simulink model "MATLAB02"  (R2023a)
settings: Solver=VariableStepAuto  StartTime=0.0  StopTime=0.1  RelTol=1e-3
libraries: spsCurrentMeasurementLib x3, spsControlledCurrentSourceLib x2, spsSeriesRLCBranchLib x2, spsDCVoltageSourceLib x1, sps_lib x1
settings Model: Creator=吉禹畅  LastModifiedBy=吉禹畅

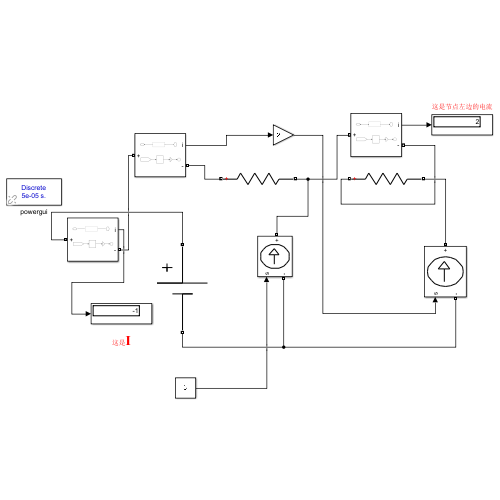
[thumbnail: Simulink's stored preview of the top-level diagram]
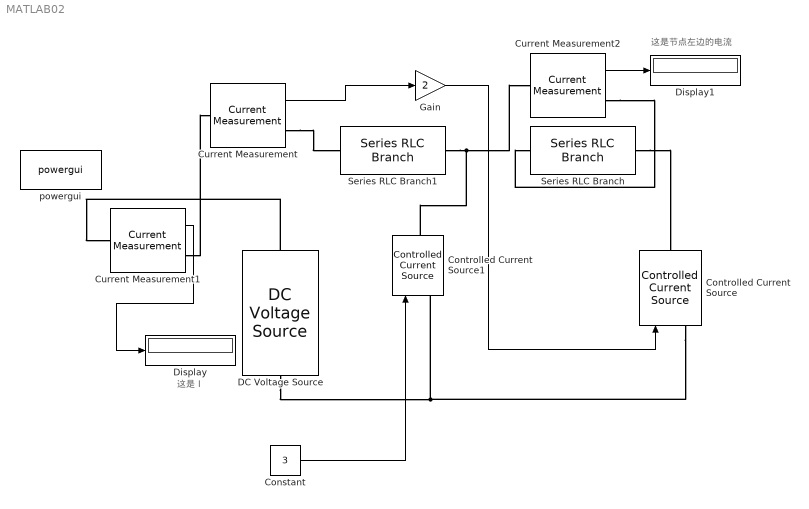
== system MATLAB02 ==
  note: 这是节点左边的电流
  note: 这是 I
  Constant : Constant  Value=3
  Controlled Current Source : spsControlledCurrentSourceLib/Controlled Current Source  Initialize=on  Source_Type=DC  Amplitude=0  Phase=0  Frequency=0  Measurements=None
  Controlled Current Source1 : spsControlledCurrentSourceLib/Controlled Current Source  Initialize=on  Source_Type=DC  Amplitude=3  Phase=0  Frequency=0  Measurements=None
  Current Measurement : spsCurrentMeasurementLib/Current Measurement  PhasorSimulation=off  OutputType=Complex  PSBequivalent=0
  Current Measurement1 : spsCurrentMeasurementLib/Current Measurement  PhasorSimulation=off  OutputType=Complex  PSBequivalent=0
  Current Measurement2 : spsCurrentMeasurementLib/Current Measurement  PhasorSimulation=off  OutputType=Complex  PSBequivalent=0
  DC Voltage Source : spsDCVoltageSourceLib/DC Voltage Source  Amplitude=10  Measurements=None
  Display : Display
  Display1 : Display
  Gain : Gain  Gain=2
  Series RLC Branch : spsSeriesRLCBranchLib/Series RLC Branch  LConnTagsString=__new0  RConnTagsString=__new0  BranchType=R  Resistance=1  Inductance=1e-3  SetiL0=off  InitialCurrent=0  Capacitance=1e-6  Setx0=off  InitialVoltage=0  Measurements=None
  Series RLC Branch1 : spsSeriesRLCBranchLib/Series RLC Branch  LConnTagsString=__new0  RConnTagsString=__new0  BranchType=R  Resistance=2  Inductance=1e-3  SetiL0=off  InitialCurrent=0  Capacitance=1e-6  Setx0=off  InitialVoltage=0  Measurements=None
  powergui : sps_lib/powergui  Priority=1  SimulationMode=Discrete  SampleTime=50e-6  frequency=60  Iterations=50  frequencyindice=0  Pbase=100e6  ErrMax=1e-4  UnitsV=kV  UnitsW=MW  buscounter=0  FunctionMessages=off  echomessages=off  EnableUseOfTLC=off  CurrentSourceSwitches=off  DisableSnubberDevices=off  DisableRonSwitches=off  DisableVfSwitches=off  DisplayEquations=off  AutomaticDiscreteSolvers=off  SolverType=Tustin/Backward Euler (TBE)  Interpol=off  ExternalGateDelay=off  methode=off  Ts=100  x0status=blocks  SPID=on  SwTol=0  HookPort=off  NonlinearTolerance=1e-4  nMaxIteration=100  ContinueOnMaxIteration=off  RestoreLinks=warning  ResistiveCurrentMeasurement=off  Frange=[0:2:500]  Ylog=off  Xlog=on  ShowGrid=off  save=off  variable=ZData  structure=0  ZoomFFT=off  StartTime=0.0  cycles=1  DisplayStyle=1  fundamental=60  FreqAxis=off  MaxFrequency=1000  frequencyindicesteady=1  RmsSteady=1  display=off
  wires:
  Current Measurement/1 -> Gain/1
  Gain/1 -> Controlled Current Source/1
  Current Measurement1/1 -> Display/1
  Current Measurement2/1 -> Display1/1
  Constant/1 -> Controlled Current Source1/1
  connections:
  Series RLC Branch1/RConn1 -- Controlled Current Source1/RConn1 -- Current Measurement2/LConn1
  DC Voltage Source/RConn1 -- Current Measurement1/LConn1
  Series RLC Branch/RConn1 -- Controlled Current Source/RConn1
  Current Measurement/RConn1 -- Series RLC Branch1/LConn1
  Current Measurement1/RConn1 -- Current Measurement/LConn1
  Current Measurement2/RConn1 -- Series RLC Branch/LConn1
  DC Voltage Source/LConn1 -- Controlled Current Source/LConn1 -- Controlled Current Source1/LConn1
